simulink model "ControlSystem"  (R2021b)
settings: Solver=VariableStepAuto  StartTime=0.0  StopTime=20  RelTol=1e-3
values from neighbouring files (symbols this model uses):
  A = 4.9e-8    (= 4.9e-08)    [init.m]
  b_s = 0.5    [init.m]
  I = 2.7e-6    (= 2.7e-06)    [init.m]
  k_s = 0.0018    [init.m]
  r = 7.5e-3    (= 0.0075)    [init.m]
settings Model: Creator=Raj Shah  LastModifiedBy=Raj Shah

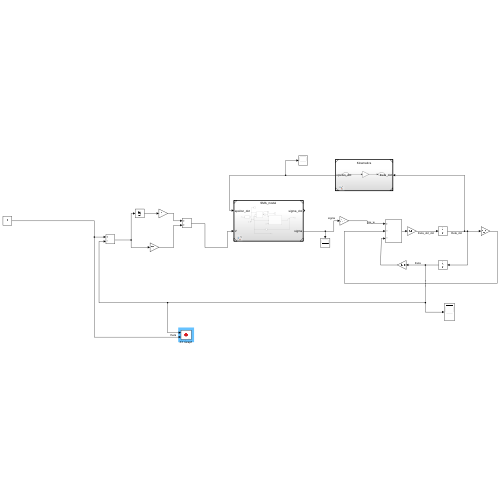
[thumbnail: Simulink's stored preview of the top-level diagram]
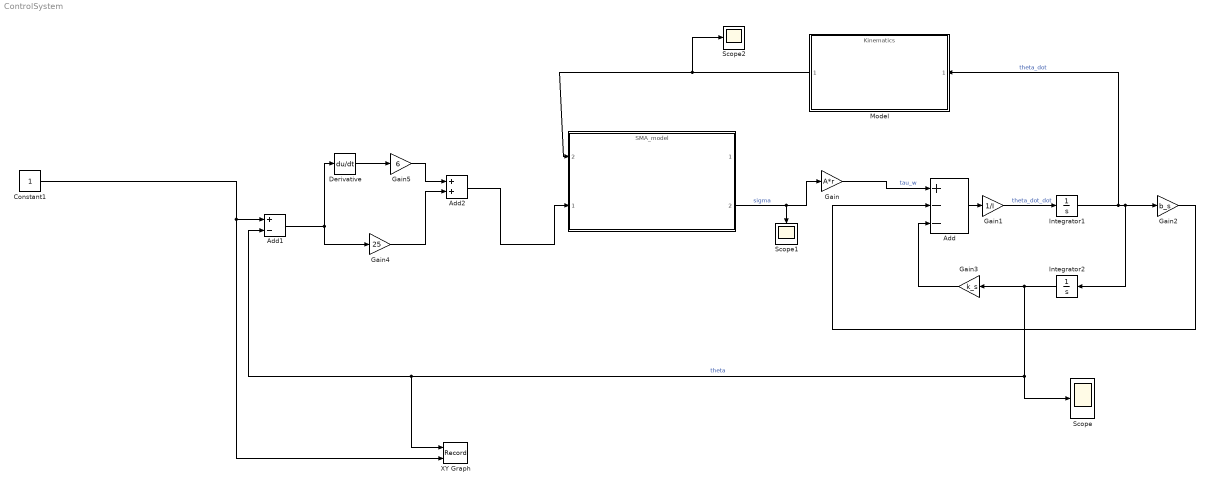
== system ControlSystem ==
  " " : ModelReference  ModelNameDialog=SMA_model.slx  SimulationMode=Normal  ModelReferenceVersion=1.40
      settings: PortSchema="{\"entries\":[{\"content\":{\"sides\":[{\"content\":{\"connectorIds\":[\"In2\",\"In1\"]},\"type\":\"ConnectorPlacement.EquallySpacedRectSide\",\"uuid\":\"608ed256-bf4a-4468-aaa6-41a0901fe41c\"},{\"content\":{\"connectorIds\":[\"Out1\",\"Out2\"],\"side\":\"RIGHT\"},\"type\":\"ConnectorPlacement.EquallySpacedRectSide\",\"uuid\":\"ea926bb8-49f4-4647-b1e1-2602f3a83e1c\"},{\"content\":{\"connectorIds\":[],\"side\":\"TOP\"},\"type\":\"ConnectorPlacement.EquallySpacedRectSide\",\"uuid\":\"2990464a-009d-4220-9d5a-e567065e0ad2\"}]},\"type\":\"ConnectorPlacement.EquallySpacedConnector\",\"uuid\":\"de33bc14-3798-4fc1-9250-22d458448bf7\"}],\"packageUris\":[\"http://schema.mathworks.com/mf0/Connector/R2020b\"],\"version\":\"1.0\"}"
  Add : Sum  Inputs=+--
  Add1 : Sum  Inputs=+-
  Add2 : Sum
  Constant1 : Constant
  Derivative : Derivative
  Gain : Gain  Gain=A*r
  Gain1 : Gain  Gain=1/I
  Gain2 : Gain  Gain=b_s
  Gain3 : Gain  Gain=k_s
  Gain4 : Gain  Gain=25
  Gain5 : Gain  Gain=6
  Integrator1 : Integrator
  Integrator2 : Integrator
  Model : ModelReference  ModelNameDialog=Kinematics.slx  SimulationMode=Normal  ModelReferenceVersion=1.1
  Scope : Scope
  Scope1 : Scope
  Scope2 : Scope
  XY Graph : Record  FileSettingsInternal="{\"entries\":[{\"content\":{\"excelSettings\":{\"content\":{},\"type\":\"Streamout.ExcelSettings\"}},\"type\":\"Streamout.FileSettingStorage\",\"uuid\":\"f417bd37-b425-422f-aa04-5c235f8087f5\"}],\"packageUris\":[\"http://schema.mathworks.com/mf0/streamout_blocks/R2020a\"],\"version\":\"1.0\"}"  Layout=[1 1]  SignalsInternal="{\"entries\":[{\"content\":{\"signals\":[{\"content\":{\"blockPath\":[\"ControlSystem/XY Graph\"],\"channel\":[],\"dimensions\":[1],\"domain\":\"ControlSystem/XY Graph\",\"lineColor\":\"#a2142f\",\"plots\":[1],\"port\":1,\"sid\":[\"\"],\"signalID\":36475,\"signalName\":\"theta\"},\"type\":\"RecordBlkView.Signal\",\"uuid\":\"fe2129fe-4ae2-4dfe-bd99-cac5433b5640\"},{\"content\":{\"blockPath\":[\"ControlSystem/XY Graph\"],\"channel\":[],\"dimensions\":[1],\"domain\":\"ControlSystem/XY Graph\",\"lineColor\":\"#139fff\",\"plots\":[1],\"port\":2,\"sid\":[\"\"],\"signalID\":36479,\"signalName\":\"Constant1\"},\"type\":\"RecordBlkView.Signal\",\"uuid\":\"ad4ac7c9-037e-495f-8849-2f4c1a200efb\"}]},\"type\":\"RecordBlkView.InputSignals\",\"uuid\":\"08e95909-470f-4458-a826-e4bd12301796\"}],\"packageUris\":[\"http://schema.mathworks.com/mf0/streamout_blocks/R2020a\"],\"version\":\"1.0\"}"  CompatibilityTag=XY
  wires:
  Add/1 -> Gain1/1
  Integrator1/1 -> Integrator2/1, Gain2/1, Model/1  "theta_dot"
  Gain2/1 -> Add/2
  Gain3/1 -> Add/3
  Integrator2/1 -> XY Graph/1, Add1/2, Scope/1, Gain3/1  "theta"
  Gain/1 -> Add/1  "tau_w"
  Model/1 -> Scope2/1, " "/2
  " "/2 -> Scope1/1, Gain/1  "sigma"
  Gain1/1 -> Integrator1/1  "theta_dot_dot"
  Constant1/1 -> XY Graph/2, Add1/1
  Add1/1 -> Gain4/1, Derivative/1
  Derivative/1 -> Gain5/1
  Gain5/1 -> Add2/1
  Gain4/1 -> Add2/2
  Add2/1 -> " "/1
